simulink model "Synchronous_Machine_Expt5"  (R2021a)
settings: Solver=ode23tb  StartTime=0.0  StopTime=inf  FixedStep=1e-3  RelTol=1e-4
libraries: spsFourierLib x3, fl_lib x3, nesl_utility x3, spsSimplifiedSynchronousMachineSIUnitsLib x1, spsThreePhaseParallelRLCLoadLib x1, spsThreePhaseProgrammableVoltageSourceLib x1, spsPower3phInstantaneousLib x1, spsThreePhaseVIMeasurementLib x1, spsGroundLib x1, spspowerguiLib x1
settings Model: ExtModeTrigMode=oneshot  ExtModeArmWhenConnect=off  ExtModeAutoUpdateStatusClock=off  Creator=MathWorks  LastModifiedBy=geoko
settings SolverCC: ZeroCrossAlgorithm=Adaptive  AlgebraicLoopSolver=TrustRegion
settings DataIOCC: InitialState=xinit  SaveFormat=Array  SignalLoggingSaveFormat=ModelDataLogs  SaveOutput=off  ReturnWorkspaceOutputs=off  TimeSaveName=t  SignalLoggingName=sigsOut
settings OptimizationCC: BooleanDataType=off  ExpressionDepthLimit=2147483647  InitFltsAndDblsToZero=on  EfficientMapNaN2IntZero=off  LifeSpan=inf
settings DebuggingCC: SaveWithParameterizedLinksMsg=none  UnderspecifiedInitializationDetection=Classic  MergeDetectMultiDrivingBlocksExec=none  SignalResolutionControl=TryResolveAllWithWarning  MultiTaskDSMMsg=warning  MultiTaskCondExecSysMsg=none  SigSpecEnsureSampleTimeMsg=none  FcnCallInpInsideContextMsg=warning  UnconnectedInputMsg=none  UnconnectedOutputMsg=none  StateNameClashWarn=warning  SFUnexpectedBacktrackingDiag=warning  SFNoUnconditionalDefaultTransitionDiag=warning  SFExecutionAtInitializationDiag=none  SFMachineParentedDataDiag=warning  ArithmeticOperatorsInVariantConditions=warning
settings HardwareCC: ProdBitPerPointer=32  ProdBitPerSizeT=32  ProdBitPerPtrDiffT=32  ProdLargestAtomicFloat=None  ProdIntDivRoundTo=Undefined  ProdEndianess=Unspecified  ProdWordSize=32  ProdHWDeviceType=32-bit Generic  TargetUnknown=on
settings ModelReferenceCC: PropagateSignalLabelsOutOfModel=off
settings SFSimCC: SimUseLocalCustomCode=off  CustomCodeUndefinedFunction=UseInterfaceOnly
settings RTWCC: Description=Generic Real-Time Target  RTWUseLocalCustomCode=off
settings CodeAppCC: StateflowObjectComments=on
settings GRTTargetCC: TargetFcnLib=ansi_tfl_tmw.mat  TargetLangStandard=C89/C90 (ANSI)  CombineOutputUpdateFcns=off  GRTInterface=on
settings ConfigComp: CovMetricSettings=dw  CovSaveCumulativeToWorkspaceVar=on  CovSaveSingleToWorkspaceVar=on  CovExternalEMLEnable=off  CovSFcnEnable=off
settings SimscapeCC: SimscapeNormalizeSystem=off

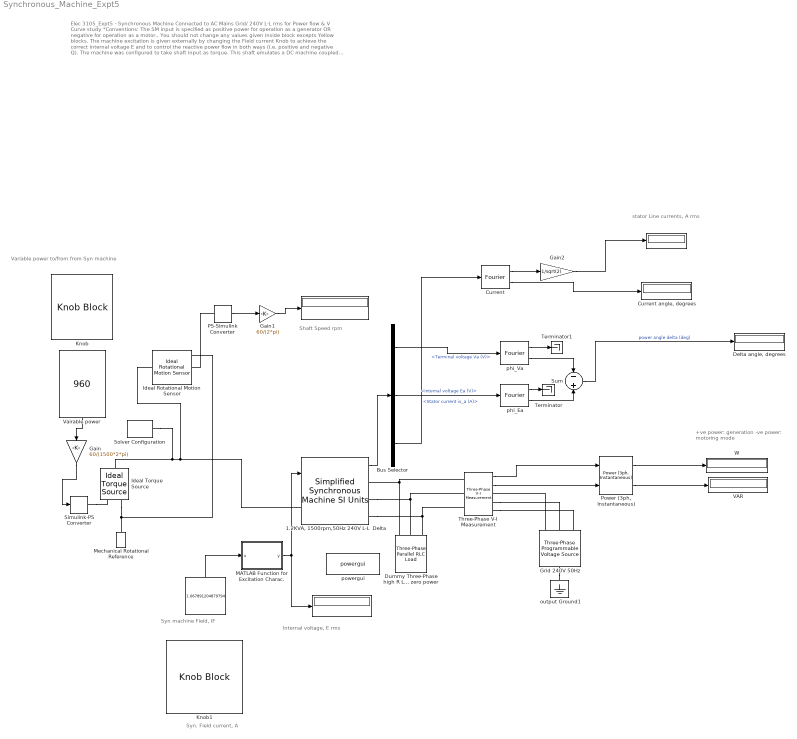
== system Synchronous_Machine_Expt5 ==
  note: Internal voltage, E rms
  note: Syn machine Field, IF
  note: Shaft Speed rpm
  note: Elec 3105_Expt5 - Synchronous Machine Connected to AC Mains Grid/ 240V L-L rms for Power flow & V Curve study
      |
      | *Conventions: The SM input is specified as positive power for operation as a generator OR negative for operation as a motor..
      | You should not change any values given inside block excepts Yellow blocks.
      | The machine excitation is given externally by changing the Field current Knob to achieve the correct internal voltage E and to control the reactive power flow in both ways (i.e. positive and negative Q).
      | The machine was configured to take shaft input as torque.
      | This shaft emulates a DC machine coupled mechanically to the Synchronous Machine similar to the experimental setup.
      | By specifying the shaft power and in turn converting into torque, as required (model by a Ideal Torque source), the Synchronous Machine is able to operate either in Motor or Generator mode.
      | Since the machine is electrically connected to the Grid, the shaft speed is fixed according to the grid frequency.
      |
      | Field current "IF" and Mechanical power values input to the respective blocks should be within boundaries (0.35 < IF <1.4, and -1000 <Pm < 960) and after running the simulation, you can observe the waveforms in the scopes
      | For stable steady-state results of the required data, avoid measurements during the initial transients by waiting for few seconds.
      | Any unstable/oscillatory waveform should be discarded; Rerun the simulation with new values of inputs (within the ranges) for the Yellow Blocks.
      | Note: The simulation is running with a stop time of inf. The simulation will run until you stop the simulation so you take all measurements in one continuous simulation.
  note: Syn. Field current, A
  note: Variable power to/from from Syn machine
  note: stator Line currents, A rms
  note: +ve power: generation
      | -ve power: motoring mode
  " " : Display
  " " : Display
  " " : Display
  " " : Constant  Value=1.067891204879794  OutMin=[0.35]  OutMax=[1.4]  OutDataTypeStr=double
  "1.2KVA, 1500rpm,50Hz 240V L-L  Delta" : spsSimplifiedSynchronousMachineSIUnitsLib/Simplified Synchronous Machine SI Units  ConnectionType=3-wire Y  MechanicalLoad=Mechanical rotational port  MeasurementBus=off  NominalParameters=[ 1200, 240, 50 ]  Mechanical="[0.03,  20,  2]"  InternalRL=[ 4.2 ,35/314]  InitialConditions=[0 3.45388 0.340207 0.340207 0.340207 0 -120 120]  IterativeDiscreteModel=Trapezoidal non iterative  TsBlock=-1  TsPowergui=0  LoadFlowParameters=[1 100 240 0 0]  Units=1  BusType=PV  Pref=0  Qref=0  Qmin=-inf  Qmax=+inf  PLF=0  QLF=0
      settings: AttributesFormatString=\n  SourceProductBaseCode=PS
  Bus Selector : BusSelector  OutputSignals=Terminal voltage Va (V),Internal voltage Ea (V),Stator current is_a (A)
  "Current " : spsFourierLib/Fourier  Freq=50  n=1  InInit=[0, 0]  Ts=0
      settings: SourceProductBaseCode=PS
  "Current angle, degrees" : Display
  "Delta angle, degrees" : Display
  "Dummy Three-Phase high R Load for system stability, consume near zero power" : spsThreePhaseParallelRLCLoadLib/Three-Phase Parallel RLC Load  LConnTagsString=A|B|C  Configuration=Y (grounded)  NominalVoltage=240  Vabc=[1e3 1e3 1e3]  Vabcp=[1e3 1e3 1e3]  NominalFrequency=50  UnbalancedPower=off  ActivePower=5  InductivePower=0  CapacitivePower=0  Pabc=[10e3 9e3 11e3]  QLabc=[100 90 110]  QCabc=[100 90 110]  Pabcp=[10e3 9e3 11e3]  QLabcp=[100 90 110]  QCabcp=[100 90 110]  Measurements=None  LoadType=constant Z
  Gain : Gain  Gain=60/(1500*2*pi)
  Gain1 : Gain  Gain=60/(2*pi)
  Gain2 : Gain  Gain=1/sqrt(2)
  Grid 240V 50Hz : spsThreePhaseProgrammableVoltageSourceLib/Three-Phase Programmable Voltage Source  PositiveSequence=[240 0 50]  VariationEntity=None  VariationType=Step  VariationTypeAlt=Step  VariationStep=-0.5  VariationRate=10  VariationMagnitude=0.3  VariationFrequency=2  VariationTiming=[0.1 1.2]  VariationPhaseA=off  Amplitudes=[1 0.8 1.2 1.0]  TimeValues=[0 0.1 0.15 0.2]  HarmonicGeneration=off  HarmonicA=[3 0.2 -25 0]  HarmonicB="[2 0.15  35 2]"  Timing="[0.05  3]"  BusType=swing  Pref=0  Qref=0  Qmin=-inf  Qmax=inf
  Ideal Rotational Motion Sensor : fl_lib/Mechanical/Mechanical Sensors/Ideal Rotational Motion Sensor  wrap_angle=simscape.enum.onoff.off  offset=0 rad
  Ideal Torque Source : fl_lib/Mechanical/Mechanical Sources/Ideal Torque Source
  Knob : KnobBlock  ScaleMin=-1000  ScaleMax=960
  Knob1 : KnobBlock  ScaleMin=0.34999999999999998  ScaleMax=1.3999999999999999
  MATLAB Function for Excitation Charac. : MATLAB Function  TreatAsAtomicUnit=on
  Mechanical Rotational Reference : fl_lib/Mechanical/Rotational Elements/Mechanical Rotational Reference
  PS-Simulink Converter : nesl_utility/PS-Simulink Converter  PhysicalDomain=network_engine_domain  SubClassName=ps_output  LeftPortType=input  RightPortType=output  PseudoPeriodic=off  Frequencies=[]  Unit=1  AffineConversion=off
      settings: SourceProductBaseCode=PW,SS
  "Power (3ph, Instantaneous)" : spsPower3phInstantaneousLib/Power (3ph, Instantaneous)
  Simulink-PS Converter : nesl_utility/Simulink-PS Converter  PhysicalDomain=network_engine_domain  SubClassName=ps_input  LeftPortType=input  RightPortType=output  PseudoPeriodic=off  Frequencies=[]  NoiseDistribution=none  NoiseParameters=[]  Unit=1  AffineConversion=off  FilteringAndDerivatives=filter  SimscapeFilterOrder=1  InputFilterTimeConstant=0.001  UdotUserProvided=1
      settings: SourceProductBaseCode=PW,SS
  Solver Configuration : nesl_utility/Solver Configuration  PhysicalDomain=network_engine_domain  SubClassName=solver  LeftPortType=input  RightPortType=generic  Tones=[]  Harmonics=[]  SimulateNoise=off  Profile=off  UseLocalSampling=off  EnableSwitchedLinearOptims=on  FrequencyDomain=off  UseCCode=off  RelTol=0.001  AbsTol=1e-06  MinStep=1e-09  ToWorkspace=off  RevertToSquareIcSolve=off  NumHomotopyIterations=100  PhasorMode=off  PhasorModeNumHarmonics=1  DoDC=off  ResidualTolerance=1e-09  UseLocalSolver=off  LocalSolverChoice=NE_BACKWARD_EULER_ADVANCER  LocalSolverSampleTime=0.001  DoFixedCost=off  MaxNonlinIter=3  MaxModeIter=2  ComputeImpulses=off  ImpulseIterations=2  LinearAlgebra=Sparse  EquationFormulation=NE_TIME_EF  DelaysMemoryBudget=1024  AutomaticFiltering=on  FilteringTimeConstant=0.001  PartitionStorageMethod=AS_NEEDED  PartitionMemoryBudget=1024  PartitionMethod=FAST
      settings: SourceProductBaseCode=PW,SS
  Sum : Sum  Inputs=-+  InputSameDT=on  SaturateOnIntegerOverflow=on  OutDataTypeStr=Inherit: Same as first input
  Terminator : Terminator
  Terminator1 : Terminator
  Three-Phase V-I Measurement : spsThreePhaseVIMeasurementLib/Three-Phase V-I Measurement  VoltageMeasurement=phase-to-ground  SetLabelV=off  LabelV=Vabc  Vpu=off  VpuLL=off  CurrentMeasurement=yes  SetLabelI=off  LabelI=Iabc  Ipu=off  Pbase=1000e6  Vbase=315e3  OutputType=Complex  PhasorSimulation=off  PSBequivalent=0
  VAR : Display
  "Vairable power " : Constant  Value=960  OutMin=[-1000]  OutMax=[960]
  W : Display
  output Ground1 : spsGroundLib/Ground  LConnTagsString=a
  phi_Ea : spsFourierLib/Fourier  Freq=50  n=1  InInit=[0, 0]  Ts=0
      settings: SourceProductBaseCode=PS
  phi_Va : spsFourierLib/Fourier  Freq=50  n=1  InInit=[0, 0]  Ts=0
      settings: SourceProductBaseCode=PS
  powergui : spspowerguiLib/powergui  Priority=2  SimulationMode=Discrete  SampleTime=100e-6  frequency=50  Iterations=50  frequencyindice=50  Pbase=1e3  ErrMax=1e-4  UnitsV=V  UnitsW=W  buscounter=0  FunctionMessages=off  echomessages=off  EnableUseOfTLC=on  CurrentSourceSwitches=off  DisableSnubberDevices=off  DisableRonSwitches=off  DisableVfSwitches=off  DisplayEquations=off  AutomaticDiscreteSolvers=off  SolverType=Tustin/Backward Euler (TBE)  Interpol=on  ExternalGateDelay=off  methode=off  Ts=0  x0status=blocks  SPID=off  SwTol=0  HookPort=off  NonlinearTolerance=1e-4  nMaxIteration=100  ContinueOnMaxIteration=off  RestoreLinks=warning  ResistiveCurrentMeasurement=off  Frange=[0:2:500]  Ylog=off  Xlog=off  ShowGrid=off  save=off  variable=ZData  structure=0  ZoomFFT=on  StartTime=0.0  cycles=1  DisplayStyle=off  fundamental=60  FreqAxis=off  MaxFrequency=1000  frequencyindicesteady=1  RmsSteady=1  display=off
  wires:
  phi_Va/2 -> Sum/1
  phi_Ea/2 -> Sum/2
  Sum/1 -> "Delta angle, degrees"/1  "power angle delta (deg)"
  "1.2KVA, 1500rpm,50Hz 240V L-L  Delta"/1 -> Bus Selector/1
  Bus Selector/1 -> phi_Va/1  "<Terminal voltage Va (V)>"
  Bus Selector/2 -> phi_Ea/1  "<Internal voltage Ea (V)>"
  Three-Phase V-I Measurement/1 -> "Power (3ph, Instantaneous)"/1
  "Power (3ph, Instantaneous)"/2 -> VAR/1
  Three-Phase V-I Measurement/2 -> "Power (3ph, Instantaneous)"/2
  Bus Selector/3 -> "Current "/1  "<Stator current is_a (A)>"
  phi_Ea/1 -> Terminator/1
  phi_Va/1 -> Terminator1/1
  "Current "/1 -> Gain2/1
  "Power (3ph, Instantaneous)"/1 -> W/1
  " "/1 -> MATLAB Function for Excitation Charac./1(u)
  Gain2/1 -> " "/1
  MATLAB Function for Excitation Charac./1(y) -> "1.2KVA, 1500rpm,50Hz 240V L-L  Delta"/1, " "/1
  Gain/1 -> Simulink-PS Converter/1
  "Vairable power "/1 -> Gain/1
  Gain1/1 -> " "/1
  PS-Simulink Converter/1 -> Gain1/1
  "Current "/2 -> "Current angle, degrees"/1
  connections:
  "Dummy Three-Phase high R Load for system stability, consume near zero power"/LConn1 -- Three-Phase V-I Measurement/LConn1 -- "1.2KVA, 1500rpm,50Hz 240V L-L  Delta"/RConn1
  Grid 240V 50Hz/RConn1 -- Three-Phase V-I Measurement/RConn1
  "1.2KVA, 1500rpm,50Hz 240V L-L  Delta"/RConn2 -- Three-Phase V-I Measurement/LConn2 -- "Dummy Three-Phase high R Load for system stability, consume near zero power"/LConn2
  "1.2KVA, 1500rpm,50Hz 240V L-L  Delta"/RConn3 -- Three-Phase V-I Measurement/LConn3 -- "Dummy Three-Phase high R Load for system stability, consume near zero power"/LConn3
  Three-Phase V-I Measurement/RConn2 -- Grid 240V 50Hz/RConn2
  Three-Phase V-I Measurement/RConn3 -- Grid 240V 50Hz/RConn3
  Grid 240V 50Hz/LConn1 -- output Ground1/LConn1
  Simulink-PS Converter/RConn1 -- Ideal Torque Source/RConn1
  Ideal Torque Source/LConn1 -- Solver Configuration/RConn1 -- Ideal Rotational Motion Sensor/LConn1 -- "1.2KVA, 1500rpm,50Hz 240V L-L  Delta"/LConn1
  Ideal Torque Source/RConn2 -- Ideal Rotational Motion Sensor/RConn1 -- Mechanical Rotational Reference/LConn1
  PS-Simulink Converter/LConn1 -- Ideal Rotational Motion Sensor/RConn2

== matlab function Synchronous_Machine_Expt5/MATLAB Function for Excitation Charac. ==
  data: u input; y output
function y = fcn(u)

y = 45.56*(u^3)-230.8*(u^2)+ 456.4*u-5.68;
end
